simulink model "Planta3Variante"  (Simulink 7.1)
settings: Solver=ode45  StartTime=0.0  StopTime=10.0  RelTol=1e-3
settings Model: Creator=ALUNO  LastModifiedBy=ALUNO

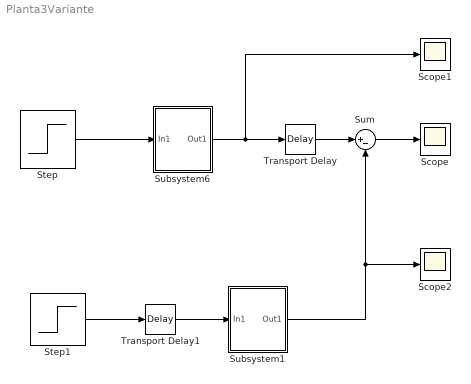
== system Planta3Variante ==
  Scope : Scope
  Scope1 : Scope
  Scope2 : Scope
      settings: SaveName=ScopeData2
  Step : Step  SampleTime=0
  Step1 : Step  SampleTime=0
  Subsystem1 : Subsystem
      mask Display: disp('Planta P3')
  Subsystem6 : Subsystem
      mask Display: disp('Planta P3')
  Sum : Sum  Inputs=|+-  OutDataType=sfix(16)  OutScaling=2^0
  Transport Delay : TransportDelay  DelayTime=3  InitialOutput=1
  Transport Delay1 : TransportDelay  DelayTime=3  InitialOutput=1
  wires:
  Step1/1 -> Transport Delay1/1
  Transport Delay1/1 -> Subsystem1/1(In1)
  Step/1 -> Subsystem6/1(In1)
  Subsystem6/1(Out1) -> Transport Delay/1, Scope1/1
  Transport Delay/1 -> Sum/1
  Subsystem1/1(Out1) -> Sum/2, Scope2/1
  Sum/1 -> Scope/1

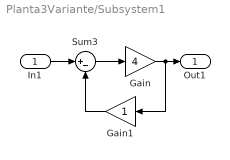
== system Planta3Variante/Subsystem1 ==
  In1 : Inport  OutDataType=sfix(16)  OutScaling=2^0
  Gain : Gain  Gain=4  ParameterDataType=sfix(16)  ParameterScaling=2^0  OutDataType=sfix(16)  OutScaling=2^0
  Gain1 : Gain  Orientation=left  ParameterDataType=sfix(16)  ParameterScaling=2^0  OutDataType=sfix(16)  OutScaling=2^0
  Sum3 : Sum  Inputs=|+-  OutDataType=sfix(16)  OutScaling=2^0
  Out1 : Outport  OutDataType=sfix(16)  OutScaling=2^0
  wires:
  In1/1 -> Sum3/1
  Gain/1 -> Gain1/1, Out1/1
  Gain1/1 -> Sum3/2
  Sum3/1 -> Gain/1

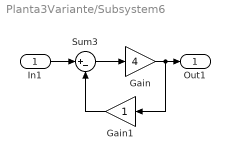
== system Planta3Variante/Subsystem6 ==
  In1 : Inport  OutDataType=sfix(16)  OutScaling=2^0
  Gain : Gain  Gain=4  ParameterDataType=sfix(16)  ParameterScaling=2^0  OutDataType=sfix(16)  OutScaling=2^0
  Gain1 : Gain  Orientation=left  ParameterDataType=sfix(16)  ParameterScaling=2^0  OutDataType=sfix(16)  OutScaling=2^0
  Sum3 : Sum  Inputs=|+-  OutDataType=sfix(16)  OutScaling=2^0
  Out1 : Outport  OutDataType=sfix(16)  OutScaling=2^0
  wires:
  In1/1 -> Sum3/1
  Gain/1 -> Gain1/1, Out1/1
  Gain1/1 -> Sum3/2
  Sum3/1 -> Gain/1
